simulink library "PQFV_lib"  (Simulink 8.1)
settings: Solver=ode45  StartTime=0.0  StopTime=10.0  RelTol=1e-3
undefined symbols (not defined in the file): cable_spec, Ts
libraries: powerlib_extras x10, cables_lib x2, PQFV_lib x1, powerlib x1
settings Model: Creator=RE25624  LastModifiedBy=re25624

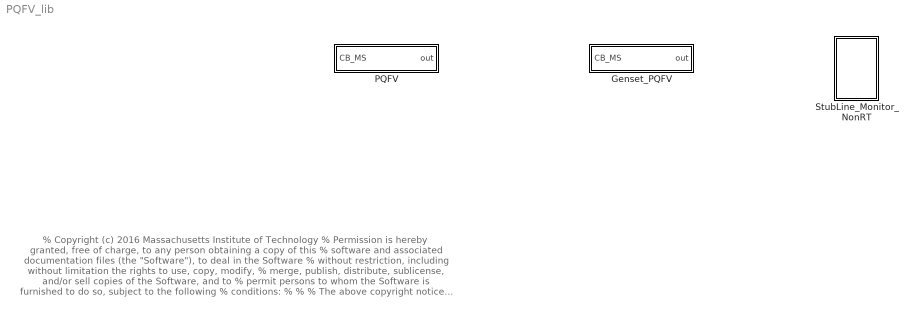
== system PQFV_lib ==
  note: % Copyright (c) 2016 Massachusetts Institute of Technology
      | % Permission is hereby granted, free of charge, to any person obtaining a copy of this
      | % software and associated documentation files (the "Software"), to deal in the Software
      | % without restriction, including without limitation the rights to use, copy, modify,
      | % merge, publish, distribute, sublicense, and/or sell copies of the Software, and to
      | % permit persons to whom the Software is furnished to do so, subject to the following
      | % conditions:
      | %
      | %
      | % The above copyright notice and this permission notice shall be included in
      | % all copies or substantial portions of the Software.
      | %
      | % THE SOFTWARE IS PROVIDED "AS IS", WITHOUT WARRANTY OF ANY KIND, EXPRESS OR IMPLIED,
      | % INCLUDING BUT NOT LIMITED TO THE WARRANTIES OF MERCHANTABILITY, FITNESS FOR A
      | % PARTICULAR PURPOSE AND NONINFRINGEMENT. IN NO EVENT SHALL THE AUTHORS OR COPYRIGHT
      | % HOLDERS BE LIABLE FOR ANY CLAIM, DAMAGES OR OTHER LIABILITY, WHETHER IN AN ACTION
      | % OF CONTRACT, TORT OR OTHERWISE, ARISING FROM, OUT OF OR IN CONNECTION WITH THE
      | % SOFTWARE OR THE USE OR OTHER DEALINGS IN THE SOFTWARE.
      | %
      | %
      | %%
  Genset_PQFV : Subsystem  mask(PQFV){VRMSLL=13800}
      mask prompts: VRMSLL "Nominal VRMSLL"
      mask help:
      | Block inputs: circuit breaker measurements
      | Block outputs: kW, kVAR, Hz, VRMSLL, Vpu, cb-status
      | -voltage as seem at the entry-point of the circuit breaker
  PQFV : Subsystem  mask(PQFV){VRMSLL=13800}
      mask prompts: VRMSLL "Nominal VRMSLL"
      mask help:
      | Block inputs: circuit breaker measurements
      | Block outputs: kW, kVAR, Hz, VRMSLL, Vpu, cb-status
      | -voltage as seem at the entry-point of the circuit breaker
  StubLine_Monitor_NonRT : Subsystem

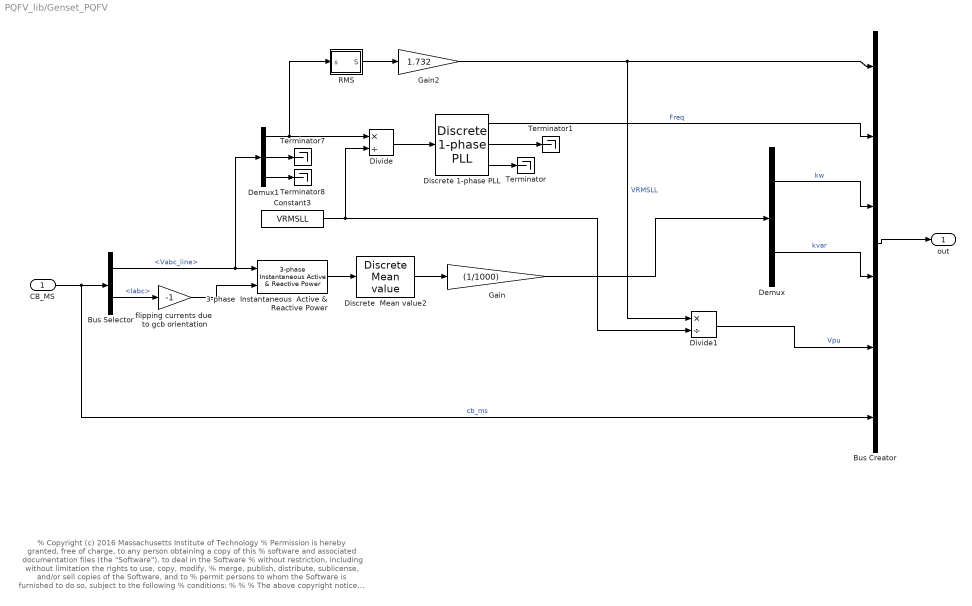
== system PQFV_lib/Genset_PQFV ==
  note: % Copyright (c) 2016 Massachusetts Institute of Technology
      | % Permission is hereby granted, free of charge, to any person obtaining a copy of this
      | % software and associated documentation files (the "Software"), to deal in the Software
      | % without restriction, including without limitation the rights to use, copy, modify,
      | % merge, publish, distribute, sublicense, and/or sell copies of the Software, and to
      | % permit persons to whom the Software is furnished to do so, subject to the following
      | % conditions:
      | %
      | %
      | % The above copyright notice and this permission notice shall be included in
      | % all copies or substantial portions of the Software.
      | %
      | % THE SOFTWARE IS PROVIDED "AS IS", WITHOUT WARRANTY OF ANY KIND, EXPRESS OR IMPLIED,
      | % INCLUDING BUT NOT LIMITED TO THE WARRANTIES OF MERCHANTABILITY, FITNESS FOR A
      | % PARTICULAR PURPOSE AND NONINFRINGEMENT. IN NO EVENT SHALL THE AUTHORS OR COPYRIGHT
      | % HOLDERS BE LIABLE FOR ANY CLAIM, DAMAGES OR OTHER LIABILITY, WHETHER IN AN ACTION
      | % OF CONTRACT, TORT OR OTHERWISE, ARISING FROM, OUT OF OR IN CONNECTION WITH THE
      | % SOFTWARE OR THE USE OR OTHER DEALINGS IN THE SOFTWARE.
      | %
      | %
      | %%
  CB_MS : Inport
  3-phase  Instantaneous  Active & Reactive Power : powerlib_extras/Measurements/3-phase  Instantaneous  Active & Reactive Power
  Bus Creator : BusCreator  Inputs=6
  Bus Selector : BusSelector  OutputSignals=Vabc_line,Iabc
  Constant3 : Constant  Value=VRMSLL
  Demux : Demux  Outputs=2
  Demux1 : Demux  Outputs=3
  Discrete 1-phase PLL : powerlib_extras/Discrete  Control Blocks/Discrete 1-phase PLL  Fmin=45  Par_Init=[0 60]  ParK=[ 180 3200 1]  Ts=Ts  AGC=on
  Discrete  Mean value2 : powerlib_extras/Discrete Measurements/Discrete  Mean value  Freq=60  Vinit=0  Ts=Ts
  Divide : Product  Inputs=*/
  Divide1 : Product  Inputs=*/
  Gain : Gain  Gain=(1/1000)
  Gain2 : Gain  Gain=1.732
  RMS : Subsystem
  Terminator{,1,7..8} (4 alike) : Terminator
  flipping currents due  to gcb orientation : Gain  Gain=-1
  out : Outport
  wires:
  flipping currents due  to gcb orientation/1 -> 3-phase  Instantaneous  Active & Reactive Power/2
  CB_MS/1 -> Bus Selector/1, Bus Creator/6  "cb_ms"
  Divide1/1 -> Bus Creator/5  "Vpu"
  Gain2/1 -> Divide1/1, Bus Creator/1  "VRMSLL"
  Bus Creator/1 -> out/1
  Bus Selector/2 -> flipping currents due  to gcb orientation/1  "<Iabc>"
  Bus Selector/1 -> 3-phase  Instantaneous  Active & Reactive Power/1, Demux1/1  "<Vabc_line>"
  Demux/2 -> Bus Creator/4  "kvar"
  Demux/1 -> Bus Creator/3  "kw"
  Discrete  Mean value2/1 -> Gain/1
  3-phase  Instantaneous  Active & Reactive Power/1 -> Discrete  Mean value2/1
  Gain/1 -> Demux/1
  Discrete 1-phase PLL/1 -> Bus Creator/2  "Freq"
  Discrete 1-phase PLL/3 -> Terminator/1
  Divide/1 -> Discrete 1-phase PLL/1
  Discrete 1-phase PLL/2 -> Terminator1/1
  Demux1/1 -> Divide/1, RMS/1(s)
  Demux1/2 -> Terminator7/1
  Demux1/3 -> Terminator8/1
  Constant3/1 -> Divide/2, Divide1/2
  RMS/1(S) -> Gain2/1

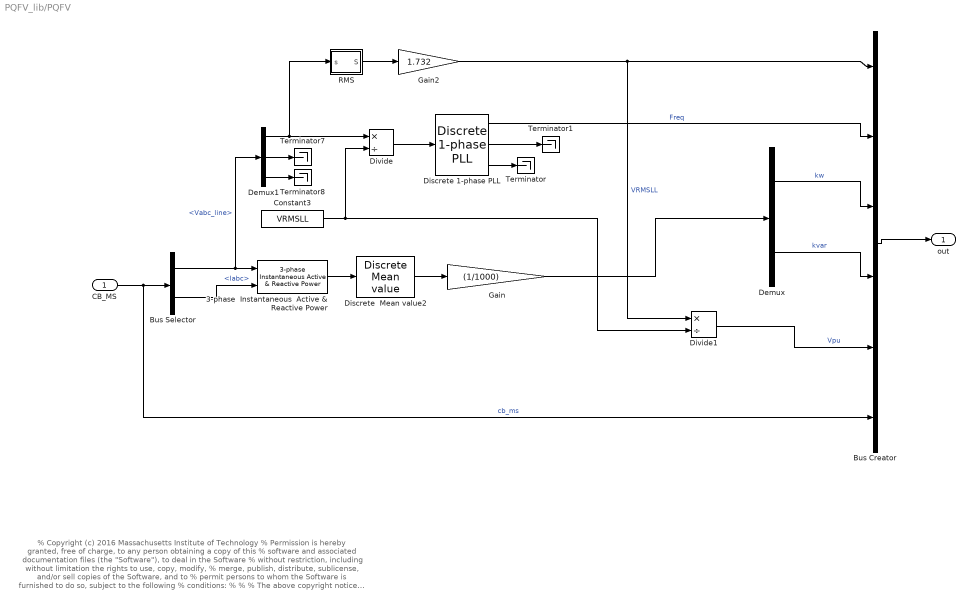
== system PQFV_lib/PQFV ==
  note: % Copyright (c) 2016 Massachusetts Institute of Technology
      | % Permission is hereby granted, free of charge, to any person obtaining a copy of this
      | % software and associated documentation files (the "Software"), to deal in the Software
      | % without restriction, including without limitation the rights to use, copy, modify,
      | % merge, publish, distribute, sublicense, and/or sell copies of the Software, and to
      | % permit persons to whom the Software is furnished to do so, subject to the following
      | % conditions:
      | %
      | %
      | % The above copyright notice and this permission notice shall be included in
      | % all copies or substantial portions of the Software.
      | %
      | % THE SOFTWARE IS PROVIDED "AS IS", WITHOUT WARRANTY OF ANY KIND, EXPRESS OR IMPLIED,
      | % INCLUDING BUT NOT LIMITED TO THE WARRANTIES OF MERCHANTABILITY, FITNESS FOR A
      | % PARTICULAR PURPOSE AND NONINFRINGEMENT. IN NO EVENT SHALL THE AUTHORS OR COPYRIGHT
      | % HOLDERS BE LIABLE FOR ANY CLAIM, DAMAGES OR OTHER LIABILITY, WHETHER IN AN ACTION
      | % OF CONTRACT, TORT OR OTHERWISE, ARISING FROM, OUT OF OR IN CONNECTION WITH THE
      | % SOFTWARE OR THE USE OR OTHER DEALINGS IN THE SOFTWARE.
      | %
      | %
      | %%
  CB_MS : Inport
  3-phase  Instantaneous  Active & Reactive Power : powerlib_extras/Measurements/3-phase  Instantaneous  Active & Reactive Power
  Bus Creator : BusCreator  Inputs=6
  Bus Selector : BusSelector  OutputSignals=Vabc_line,Iabc
  Constant3 : Constant  Value=VRMSLL
  Demux : Demux  Outputs=2
  Demux1 : Demux  Outputs=3
  Discrete 1-phase PLL : powerlib_extras/Discrete  Control Blocks/Discrete 1-phase PLL  Fmin=45  Par_Init=[0 60]  ParK=[ 180 3200 1]  Ts=Ts  AGC=on
  Discrete  Mean value2 : powerlib_extras/Discrete Measurements/Discrete  Mean value  Freq=60  Vinit=0  Ts=Ts
  Divide : Product  Inputs=*/
  Divide1 : Product  Inputs=*/
  Gain : Gain  Gain=(1/1000)
  Gain2 : Gain  Gain=1.732
  RMS : Subsystem
  Terminator{,1,7..8} (4 alike) : Terminator
  out : Outport
  wires:
  CB_MS/1 -> Bus Selector/1, Bus Creator/6  "cb_ms"
  Divide1/1 -> Bus Creator/5  "Vpu"
  Gain2/1 -> Divide1/1, Bus Creator/1  "VRMSLL"
  Bus Creator/1 -> out/1
  Bus Selector/2 -> 3-phase  Instantaneous  Active & Reactive Power/2  "<Iabc>"
  Bus Selector/1 -> 3-phase  Instantaneous  Active & Reactive Power/1, Demux1/1  "<Vabc_line>"
  Demux/2 -> Bus Creator/4  "kvar"
  Demux/1 -> Bus Creator/3  "kw"
  Discrete  Mean value2/1 -> Gain/1
  3-phase  Instantaneous  Active & Reactive Power/1 -> Discrete  Mean value2/1
  Gain/1 -> Demux/1
  Discrete 1-phase PLL/1 -> Bus Creator/2  "Freq"
  Discrete 1-phase PLL/3 -> Terminator/1
  Divide/1 -> Discrete 1-phase PLL/1
  Discrete 1-phase PLL/2 -> Terminator1/1
  Demux1/1 -> Divide/1, RMS/1(s)
  Demux1/2 -> Terminator7/1
  Demux1/3 -> Terminator8/1
  Constant3/1 -> Divide/2, Divide1/2
  RMS/1(S) -> Gain2/1

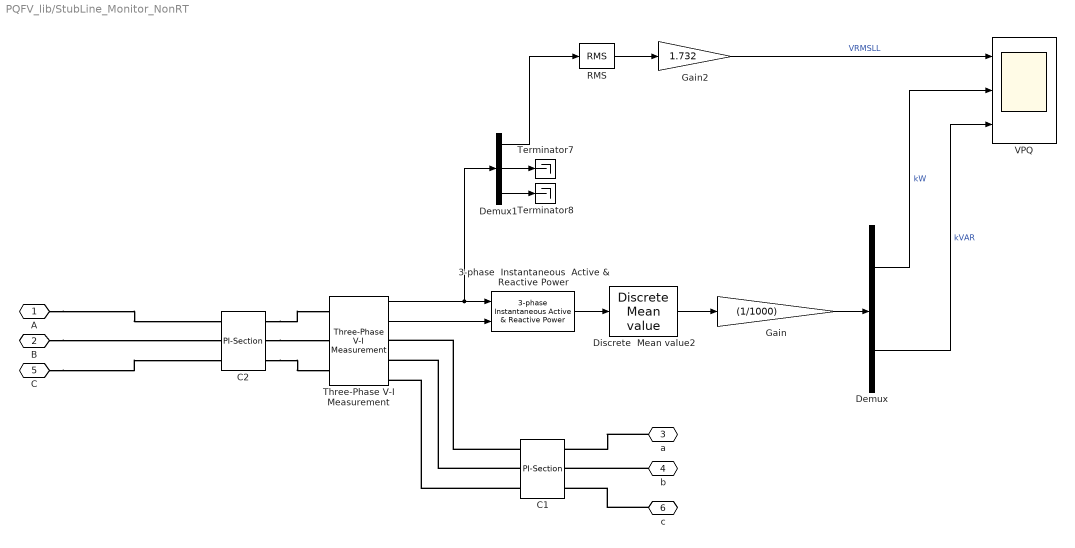
== system PQFV_lib/StubLine_Monitor_NonRT ==
  3-phase  Instantaneous  Active & Reactive Power : powerlib_extras/Measurements/3-phase  Instantaneous  Active & Reactive Power
  C1 : cables_lib/PI-Section  cable_spec=[cable_spec(13, :)]  line_length=2500  parallel_sets=1
  C2 : cables_lib/PI-Section  cable_spec=[cable_spec(13, :)]  line_length=2500  parallel_sets=1
  Demux : Demux  Outputs=2
  Demux1 : Demux  Outputs=3
  Discrete  Mean value2 : powerlib_extras/Discrete Measurements/Discrete  Mean value  Freq=60  Vinit=0  Ts=Ts
  Gain : Gain  Gain=(1/1000)
  Gain2 : Gain  Gain=1.732
  RMS : PQFV_lib/PQFV/RMS
  Terminator7 : Terminator
  Terminator8 : Terminator
  Three-Phase V-I Measurement : powerlib/Measurements/Three-Phase V-I Measurement  VoltageMeasurement=phase-to-ground  SetLabelV=off  LabelV=Vabc  Vpu=off  VpuLL=off  CurrentMeasurement=yes  SetLabelI=off  LabelI=Iabc  Ipu=off  Pbase=100e6  Vbase=500e3  OutputType=Complex  PhasorSimulation=off  PSBequivalent=0
  VPQ : Scope  NumInputPorts=3
      settings: TimeRange=0.2000000000000002  YMin=13700~13700~13700  YMax=15000~15000~15000  SaveName=ScopeData2
  A : PMIOPort  Port=1  Side=Left
  B : PMIOPort  Port=2  Side=Left
  a : PMIOPort  Port=3  Side=Right
  b : PMIOPort  Port=4  Side=Right
  C : PMIOPort  Port=5  Side=Left
  c : PMIOPort  Port=6  Side=Right
  wires:
  Gain/1 -> Demux/1
  RMS/1 -> Gain2/1
  Demux1/3 -> Terminator8/1
  Demux1/2 -> Terminator7/1
  Demux1/1 -> RMS/1
  3-phase  Instantaneous  Active & Reactive Power/1 -> Discrete  Mean value2/1
  Discrete  Mean value2/1 -> Gain/1
  Three-Phase V-I Measurement/1 -> Demux1/1, 3-phase  Instantaneous  Active & Reactive Power/1
  Three-Phase V-I Measurement/2 -> 3-phase  Instantaneous  Active & Reactive Power/2
  Gain2/1 -> VPQ/1  "VRMSLL"
  Demux/1 -> VPQ/2  "kW"
  Demux/2 -> VPQ/3  "kVAR"
  connections:
  C/RConn1 -- C2/LConn3
  A/RConn1 -- C2/LConn1
  B/RConn1 -- C2/LConn2
  C2/RConn3 -- Three-Phase V-I Measurement/LConn3
  C2/RConn1 -- Three-Phase V-I Measurement/LConn1
  C2/RConn2 -- Three-Phase V-I Measurement/LConn2
  C1/LConn2 -- Three-Phase V-I Measurement/RConn2
  C1/LConn3 -- Three-Phase V-I Measurement/RConn3
  C1/LConn1 -- Three-Phase V-I Measurement/RConn1
  c/RConn1 -- C1/RConn3
  a/RConn1 -- C1/RConn1
  b/RConn1 -- C1/RConn2

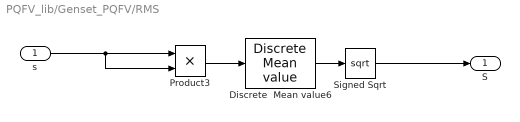
== system PQFV_lib/Genset_PQFV/RMS ==
  s : Inport
  Discrete  Mean value6 : powerlib_extras/Discrete Measurements/Discrete  Mean value  Freq=60  Vinit=0  Ts=Ts
  Product3 : Product  RndMeth=Zero
  Signed Sqrt : Sqrt  SaturateOnIntegerOverflow=on
  S : Outport
  wires:
  s/1 -> Product3/1, Product3/2
  Product3/1 -> Discrete  Mean value6/1
  Discrete  Mean value6/1 -> Signed Sqrt/1
  Signed Sqrt/1 -> S/1

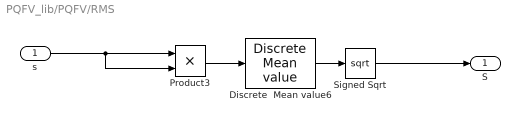
== system PQFV_lib/PQFV/RMS ==
  s : Inport
  Discrete  Mean value6 : powerlib_extras/Discrete Measurements/Discrete  Mean value  Freq=60  Vinit=0  Ts=Ts
  Product3 : Product  RndMeth=Zero
  Signed Sqrt : Sqrt  SaturateOnIntegerOverflow=on
  S : Outport
  wires:
  s/1 -> Product3/1, Product3/2
  Product3/1 -> Discrete  Mean value6/1
  Discrete  Mean value6/1 -> Signed Sqrt/1
  Signed Sqrt/1 -> S/1
